simulink model "TST_Tra_Prt"  (R2016b)
settings: Solver=FixedStepDiscrete  StartTime=0.0  StopTime=simTime  FixedStep=sampleTime  RelTol=1e-3
values from neighbouring files (symbols this model uses):
  testCase = 1    [initTST_Tra_Prt_001.m]    (also in initTST_Tra_Prt_002.m = 2; initTST_Tra_Prt_003.m = 3; initTST_Tra_Prt_004.m = 4)
libraries: simulink x9, UnitTest_Lib x4
settings Model: Creator=zhengjinyan  LastModifiedBy=zhengjinyan
settings DebuggingCC: SignalRangeChecking=error

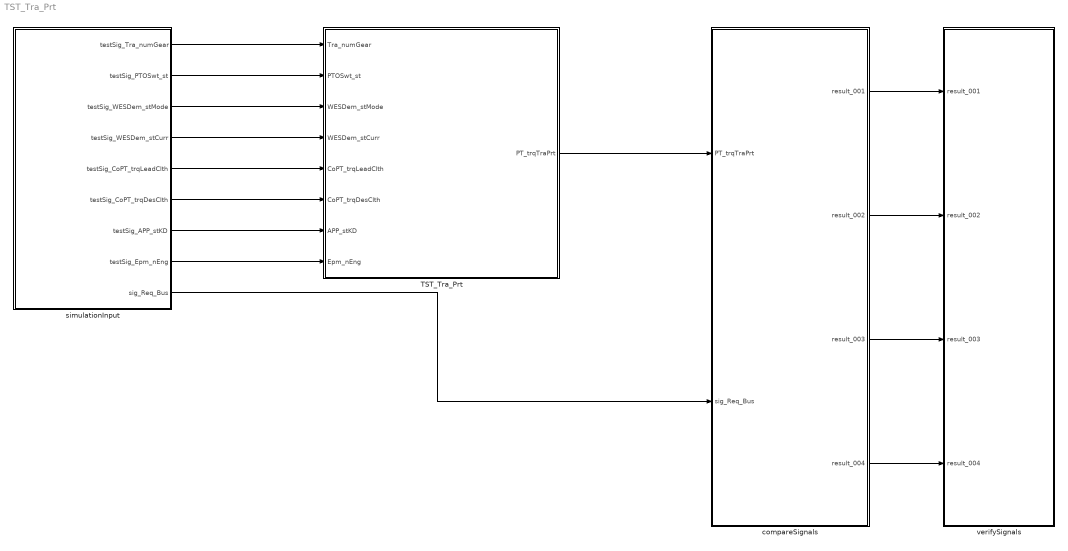
== system TST_Tra_Prt ==
  TST_Tra_Prt : Subsystem
  compareSignals : Subsystem
  simulationInput : Subsystem
  verifySignals : Subsystem
  wires:
  simulationInput/1(testSig_Tra_numGear) -> TST_Tra_Prt/1(Tra_numGear)
  simulationInput/2(testSig_PTOSwt_st) -> TST_Tra_Prt/2(PTOSwt_st)
  simulationInput/3(testSig_WESDem_stMode) -> TST_Tra_Prt/3(WESDem_stMode)
  simulationInput/4(testSig_WESDem_stCurr) -> TST_Tra_Prt/4(WESDem_stCurr)
  simulationInput/5(testSig_CoPT_trqLeadClth) -> TST_Tra_Prt/5(CoPT_trqLeadClth)
  simulationInput/6(testSig_CoPT_trqDesClth) -> TST_Tra_Prt/6(CoPT_trqDesClth)
  simulationInput/7(testSig_APP_stKD) -> TST_Tra_Prt/7(APP_stKD)
  simulationInput/8(testSig_Epm_nEng) -> TST_Tra_Prt/8(Epm_nEng)
  TST_Tra_Prt/1(PT_trqTraPrt) -> compareSignals/1(PT_trqTraPrt)
  simulationInput/9(sig_Req_Bus) -> compareSignals/2(sig_Req_Bus)
  compareSignals/1(result_001) -> verifySignals/1(result_001)
  compareSignals/2(result_002) -> verifySignals/2(result_002)
  compareSignals/3(result_003) -> verifySignals/3(result_003)
  compareSignals/4(result_004) -> verifySignals/4(result_004)

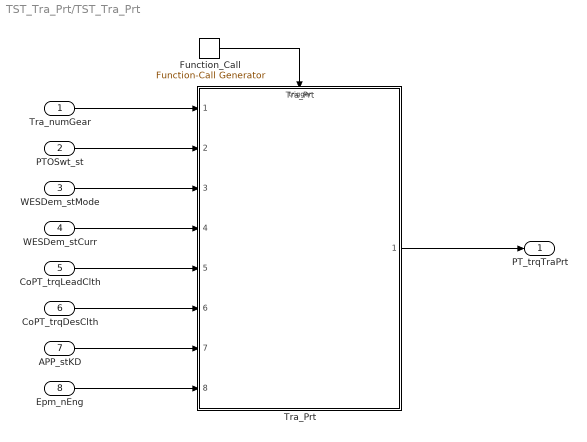
== system TST_Tra_Prt/TST_Tra_Prt ==
  Tra_numGear : Inport
  PTOSwt_st : Inport  Port=2
  WESDem_stMode : Inport  Port=3
  WESDem_stCurr : Inport  Port=4
  CoPT_trqLeadClth : Inport  Port=5
  CoPT_trqDesClth : Inport  Port=6
  APP_stKD : Inport  Port=7
  Epm_nEng : Inport  Port=8
  Function_Call : simulink/Ports & Subsystems/Function-Call Generator  sample_time=sampleTime  numberOfIterations=1
  Tra_Prt : ModelReference  ModelNameDialog=Tra_Prt  SimulationMode=Normal  ModelReferenceVersion=1.31  TriggerPortName=function  TriggerPortTriggerType=function-call  TriggerPortStatesWhenEnabling=held
  PT_trqTraPrt : Outport
  wires:
  Function_Call/1 -> Tra_Prt/Trigger
  Tra_numGear/1 -> Tra_Prt/1
  PTOSwt_st/1 -> Tra_Prt/2
  WESDem_stMode/1 -> Tra_Prt/3
  WESDem_stCurr/1 -> Tra_Prt/4
  CoPT_trqLeadClth/1 -> Tra_Prt/5
  CoPT_trqDesClth/1 -> Tra_Prt/6
  APP_stKD/1 -> Tra_Prt/7
  Epm_nEng/1 -> Tra_Prt/8
  Tra_Prt/1 -> PT_trqTraPrt/1

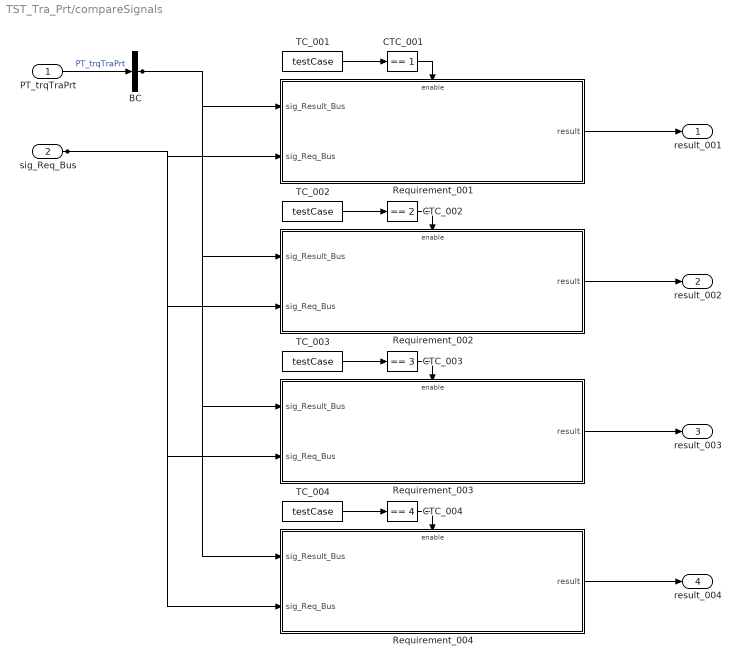
== system TST_Tra_Prt/compareSignals ==
  PT_trqTraPrt : Inport
  sig_Req_Bus : Inport  Port=2
  BC : BusCreator  Inputs=1
  CTC_001 : simulink/Logic and Bit Operations/Compare To Constant  relop===  const=1  OutDataTypeStr=boolean
  CTC_002 : simulink/Logic and Bit Operations/Compare To Constant  relop===  const=2  OutDataTypeStr=boolean
  CTC_003 : simulink/Logic and Bit Operations/Compare To Constant  relop===  const=3  OutDataTypeStr=boolean
  CTC_004 : simulink/Logic and Bit Operations/Compare To Constant  relop===  const=4  OutDataTypeStr=boolean
  Requirement_001 : Subsystem
  Requirement_002 : Subsystem
  Requirement_003 : Subsystem
  Requirement_004 : Subsystem
  TC_001 : Constant  Value=testCase
  TC_002 : Constant  Value=testCase
  TC_003 : Constant  Value=testCase
  TC_004 : Constant  Value=testCase
  result_001 : Outport
  result_002 : Outport  Port=2
  result_003 : Outport  Port=3
  result_004 : Outport  Port=4
  wires:
  PT_trqTraPrt/1 -> BC/1  "PT_trqTraPrt"
  TC_001/1 -> CTC_001/1
  CTC_001/1 -> Requirement_001/Enable
  sig_Req_Bus/1 -> Requirement_001/2(sig_Req_Bus), Requirement_002/2(sig_Req_Bus), Requirement_003/2(sig_Req_Bus), Requirement_004/2(sig_Req_Bus)
  BC/1 -> Requirement_001/1(sig_Result_Bus), Requirement_002/1(sig_Result_Bus), Requirement_003/1(sig_Result_Bus), Requirement_004/1(sig_Result_Bus)
  Requirement_001/1(result) -> result_001/1
  TC_002/1 -> CTC_002/1
  CTC_002/1 -> Requirement_002/Enable
  Requirement_002/1(result) -> result_002/1
  TC_003/1 -> CTC_003/1
  CTC_003/1 -> Requirement_003/Enable
  Requirement_003/1(result) -> result_003/1
  TC_004/1 -> CTC_004/1
  CTC_004/1 -> Requirement_004/Enable
  Requirement_004/1(result) -> result_004/1

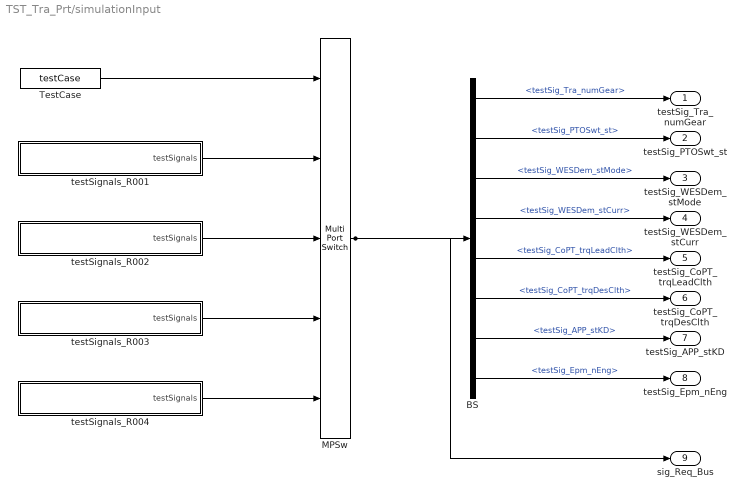
== system TST_Tra_Prt/simulationInput ==
  BS : BusSelector  OutputSignals=testSig_Tra_numGear,testSig_PTOSwt_st,testSig_WESDem_stMode,testSig_WESDem_stCurr,testSig_CoPT_trqLeadClth,testSig_CoPT_trqDesClth,testSig_APP_stKD,testSig_Epm_nEng
  MPSw : MultiPortSwitch  Inputs=4  SaturateOnIntegerOverflow=on  InputSameDT=on
  TestCase : Constant  Value=testCase
  testSignals_R001 : Subsystem
  testSignals_R002 : Subsystem
  testSignals_R003 : Subsystem
  testSignals_R004 : Subsystem
  testSig_Tra_numGear : Outport
  testSig_PTOSwt_st : Outport  Port=2
  testSig_WESDem_stMode : Outport  Port=3
  testSig_WESDem_stCurr : Outport  Port=4
  testSig_CoPT_trqLeadClth : Outport  Port=5
  testSig_CoPT_trqDesClth : Outport  Port=6
  testSig_APP_stKD : Outport  Port=7
  testSig_Epm_nEng : Outport  Port=8
  sig_Req_Bus : Outport  Port=9
  wires:
  BS/1 -> testSig_Tra_numGear/1  "<testSig_Tra_numGear>"
  BS/2 -> testSig_PTOSwt_st/1  "<testSig_PTOSwt_st>"
  BS/3 -> testSig_WESDem_stMode/1  "<testSig_WESDem_stMode>"
  BS/4 -> testSig_WESDem_stCurr/1  "<testSig_WESDem_stCurr>"
  BS/5 -> testSig_CoPT_trqLeadClth/1  "<testSig_CoPT_trqLeadClth>"
  BS/6 -> testSig_CoPT_trqDesClth/1  "<testSig_CoPT_trqDesClth>"
  BS/7 -> testSig_APP_stKD/1  "<testSig_APP_stKD>"
  BS/8 -> testSig_Epm_nEng/1  "<testSig_Epm_nEng>"
  MPSw/1 -> BS/1, sig_Req_Bus/1
  TestCase/1 -> MPSw/1
  testSignals_R001/1(testSignals) -> MPSw/2
  testSignals_R002/1(testSignals) -> MPSw/3
  testSignals_R003/1(testSignals) -> MPSw/4
  testSignals_R004/1(testSignals) -> MPSw/5

== system TST_Tra_Prt/verifySignals ==
  result_001 : Inport
  result_002 : Inport  Port=2
  result_003 : Inport  Port=3
  result_004 : Inport  Port=4
  Assertion_001 : Assertion  Enabled=off
  Assertion_002 : Assertion  Enabled=off
  Assertion_003 : Assertion  Enabled=off
  Assertion_004 : Assertion  Enabled=off
  wires:
  result_001/1 -> Assertion_001/1
  result_002/1 -> Assertion_002/1
  result_003/1 -> Assertion_003/1
  result_004/1 -> Assertion_004/1

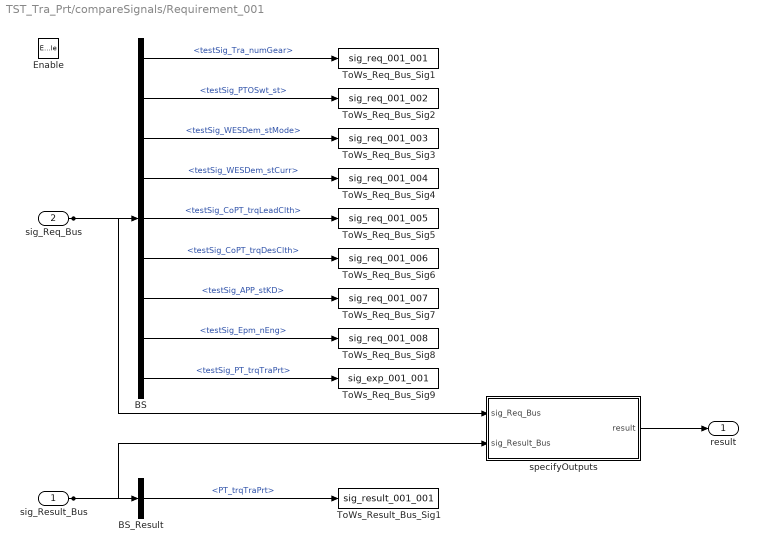
== system TST_Tra_Prt/compareSignals/Requirement_001 ==
  sig_Result_Bus : Inport
  sig_Req_Bus : Inport  Port=2
  Enable : EnablePort
  BS : BusSelector  OutputSignals=testSig_Tra_numGear,testSig_PTOSwt_st,testSig_WESDem_stMode,testSig_WESDem_stCurr,testSig_CoPT_trqLeadClth,testSig_CoPT_trqDesClth,testSig_APP_stKD,testSig_Epm_nEng,testSig_PT_trqTraPrt
  BS_Result : BusSelector  OutputSignals=PT_trqTraPrt
  ToWs_Req_Bus_Sig1 : ToWorkspace  VariableName=sig_req_001_001  SaveFormat=Structure With Time
  ToWs_Req_Bus_Sig2 : ToWorkspace  VariableName=sig_req_001_002  SaveFormat=Structure With Time
  ToWs_Req_Bus_Sig3 : ToWorkspace  VariableName=sig_req_001_003  SaveFormat=Structure With Time
  ToWs_Req_Bus_Sig4 : ToWorkspace  VariableName=sig_req_001_004  SaveFormat=Structure With Time
  ToWs_Req_Bus_Sig5 : ToWorkspace  VariableName=sig_req_001_005  SaveFormat=Structure With Time
  ToWs_Req_Bus_Sig6 : ToWorkspace  VariableName=sig_req_001_006  SaveFormat=Structure With Time
  ToWs_Req_Bus_Sig7 : ToWorkspace  VariableName=sig_req_001_007  SaveFormat=Structure With Time
  ToWs_Req_Bus_Sig8 : ToWorkspace  VariableName=sig_req_001_008  SaveFormat=Structure With Time
  ToWs_Req_Bus_Sig9 : ToWorkspace  VariableName=sig_exp_001_001  SaveFormat=Structure With Time
  ToWs_Result_Bus_Sig1 : ToWorkspace  VariableName=sig_result_001_001  SaveFormat=Structure With Time
  specifyOutputs : Subsystem
  result : Outport
  wires:
  sig_Req_Bus/1 -> BS/1, specifyOutputs/1(sig_Req_Bus)
  BS/1 -> ToWs_Req_Bus_Sig1/1  "<testSig_Tra_numGear>"
  BS/2 -> ToWs_Req_Bus_Sig2/1  "<testSig_PTOSwt_st>"
  BS/3 -> ToWs_Req_Bus_Sig3/1  "<testSig_WESDem_stMode>"
  BS/4 -> ToWs_Req_Bus_Sig4/1  "<testSig_WESDem_stCurr>"
  BS/5 -> ToWs_Req_Bus_Sig5/1  "<testSig_CoPT_trqLeadClth>"
  BS/6 -> ToWs_Req_Bus_Sig6/1  "<testSig_CoPT_trqDesClth>"
  BS/7 -> ToWs_Req_Bus_Sig7/1  "<testSig_APP_stKD>"
  BS/8 -> ToWs_Req_Bus_Sig8/1  "<testSig_Epm_nEng>"
  BS/9 -> ToWs_Req_Bus_Sig9/1  "<testSig_PT_trqTraPrt>"
  sig_Result_Bus/1 -> BS_Result/1, specifyOutputs/2(sig_Result_Bus)
  BS_Result/1 -> ToWs_Result_Bus_Sig1/1  "<PT_trqTraPrt>"
  specifyOutputs/1(result) -> result/1

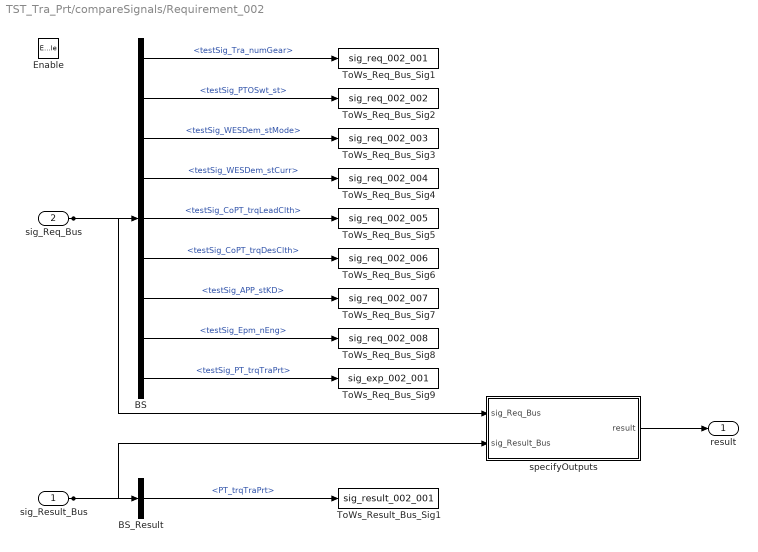
== system TST_Tra_Prt/compareSignals/Requirement_002 ==
  sig_Result_Bus : Inport
  sig_Req_Bus : Inport  Port=2
  Enable : EnablePort
  BS : BusSelector  OutputSignals=testSig_Tra_numGear,testSig_PTOSwt_st,testSig_WESDem_stMode,testSig_WESDem_stCurr,testSig_CoPT_trqLeadClth,testSig_CoPT_trqDesClth,testSig_APP_stKD,testSig_Epm_nEng,testSig_PT_trqTraPrt
  BS_Result : BusSelector  OutputSignals=PT_trqTraPrt
  ToWs_Req_Bus_Sig1 : ToWorkspace  VariableName=sig_req_002_001  SaveFormat=Structure With Time
  ToWs_Req_Bus_Sig2 : ToWorkspace  VariableName=sig_req_002_002  SaveFormat=Structure With Time
  ToWs_Req_Bus_Sig3 : ToWorkspace  VariableName=sig_req_002_003  SaveFormat=Structure With Time
  ToWs_Req_Bus_Sig4 : ToWorkspace  VariableName=sig_req_002_004  SaveFormat=Structure With Time
  ToWs_Req_Bus_Sig5 : ToWorkspace  VariableName=sig_req_002_005  SaveFormat=Structure With Time
  ToWs_Req_Bus_Sig6 : ToWorkspace  VariableName=sig_req_002_006  SaveFormat=Structure With Time
  ToWs_Req_Bus_Sig7 : ToWorkspace  VariableName=sig_req_002_007  SaveFormat=Structure With Time
  ToWs_Req_Bus_Sig8 : ToWorkspace  VariableName=sig_req_002_008  SaveFormat=Structure With Time
  ToWs_Req_Bus_Sig9 : ToWorkspace  VariableName=sig_exp_002_001  SaveFormat=Structure With Time
  ToWs_Result_Bus_Sig1 : ToWorkspace  VariableName=sig_result_002_001  SaveFormat=Structure With Time
  specifyOutputs : Subsystem
  result : Outport
  wires:
  sig_Req_Bus/1 -> BS/1, specifyOutputs/1(sig_Req_Bus)
  BS/1 -> ToWs_Req_Bus_Sig1/1  "<testSig_Tra_numGear>"
  BS/2 -> ToWs_Req_Bus_Sig2/1  "<testSig_PTOSwt_st>"
  BS/3 -> ToWs_Req_Bus_Sig3/1  "<testSig_WESDem_stMode>"
  BS/4 -> ToWs_Req_Bus_Sig4/1  "<testSig_WESDem_stCurr>"
  BS/5 -> ToWs_Req_Bus_Sig5/1  "<testSig_CoPT_trqLeadClth>"
  BS/6 -> ToWs_Req_Bus_Sig6/1  "<testSig_CoPT_trqDesClth>"
  BS/7 -> ToWs_Req_Bus_Sig7/1  "<testSig_APP_stKD>"
  BS/8 -> ToWs_Req_Bus_Sig8/1  "<testSig_Epm_nEng>"
  BS/9 -> ToWs_Req_Bus_Sig9/1  "<testSig_PT_trqTraPrt>"
  sig_Result_Bus/1 -> BS_Result/1, specifyOutputs/2(sig_Result_Bus)
  BS_Result/1 -> ToWs_Result_Bus_Sig1/1  "<PT_trqTraPrt>"
  specifyOutputs/1(result) -> result/1

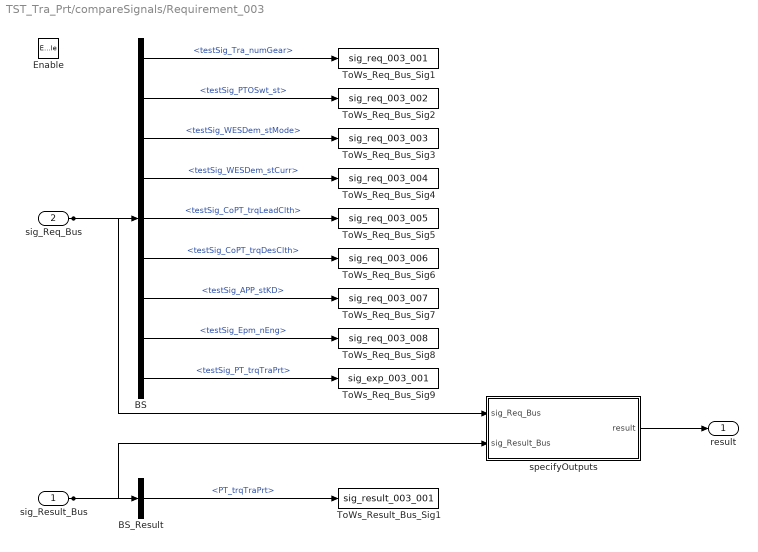
== system TST_Tra_Prt/compareSignals/Requirement_003 ==
  sig_Result_Bus : Inport
  sig_Req_Bus : Inport  Port=2
  Enable : EnablePort
  BS : BusSelector  OutputSignals=testSig_Tra_numGear,testSig_PTOSwt_st,testSig_WESDem_stMode,testSig_WESDem_stCurr,testSig_CoPT_trqLeadClth,testSig_CoPT_trqDesClth,testSig_APP_stKD,testSig_Epm_nEng,testSig_PT_trqTraPrt
  BS_Result : BusSelector  OutputSignals=PT_trqTraPrt
  ToWs_Req_Bus_Sig1 : ToWorkspace  VariableName=sig_req_003_001  SaveFormat=Structure With Time
  ToWs_Req_Bus_Sig2 : ToWorkspace  VariableName=sig_req_003_002  SaveFormat=Structure With Time
  ToWs_Req_Bus_Sig3 : ToWorkspace  VariableName=sig_req_003_003  SaveFormat=Structure With Time
  ToWs_Req_Bus_Sig4 : ToWorkspace  VariableName=sig_req_003_004  SaveFormat=Structure With Time
  ToWs_Req_Bus_Sig5 : ToWorkspace  VariableName=sig_req_003_005  SaveFormat=Structure With Time
  ToWs_Req_Bus_Sig6 : ToWorkspace  VariableName=sig_req_003_006  SaveFormat=Structure With Time
  ToWs_Req_Bus_Sig7 : ToWorkspace  VariableName=sig_req_003_007  SaveFormat=Structure With Time
  ToWs_Req_Bus_Sig8 : ToWorkspace  VariableName=sig_req_003_008  SaveFormat=Structure With Time
  ToWs_Req_Bus_Sig9 : ToWorkspace  VariableName=sig_exp_003_001  SaveFormat=Structure With Time
  ToWs_Result_Bus_Sig1 : ToWorkspace  VariableName=sig_result_003_001  SaveFormat=Structure With Time
  specifyOutputs : Subsystem
  result : Outport
  wires:
  sig_Req_Bus/1 -> BS/1, specifyOutputs/1(sig_Req_Bus)
  BS/1 -> ToWs_Req_Bus_Sig1/1  "<testSig_Tra_numGear>"
  BS/2 -> ToWs_Req_Bus_Sig2/1  "<testSig_PTOSwt_st>"
  BS/3 -> ToWs_Req_Bus_Sig3/1  "<testSig_WESDem_stMode>"
  BS/4 -> ToWs_Req_Bus_Sig4/1  "<testSig_WESDem_stCurr>"
  BS/5 -> ToWs_Req_Bus_Sig5/1  "<testSig_CoPT_trqLeadClth>"
  BS/6 -> ToWs_Req_Bus_Sig6/1  "<testSig_CoPT_trqDesClth>"
  BS/7 -> ToWs_Req_Bus_Sig7/1  "<testSig_APP_stKD>"
  BS/8 -> ToWs_Req_Bus_Sig8/1  "<testSig_Epm_nEng>"
  BS/9 -> ToWs_Req_Bus_Sig9/1  "<testSig_PT_trqTraPrt>"
  sig_Result_Bus/1 -> BS_Result/1, specifyOutputs/2(sig_Result_Bus)
  BS_Result/1 -> ToWs_Result_Bus_Sig1/1  "<PT_trqTraPrt>"
  specifyOutputs/1(result) -> result/1

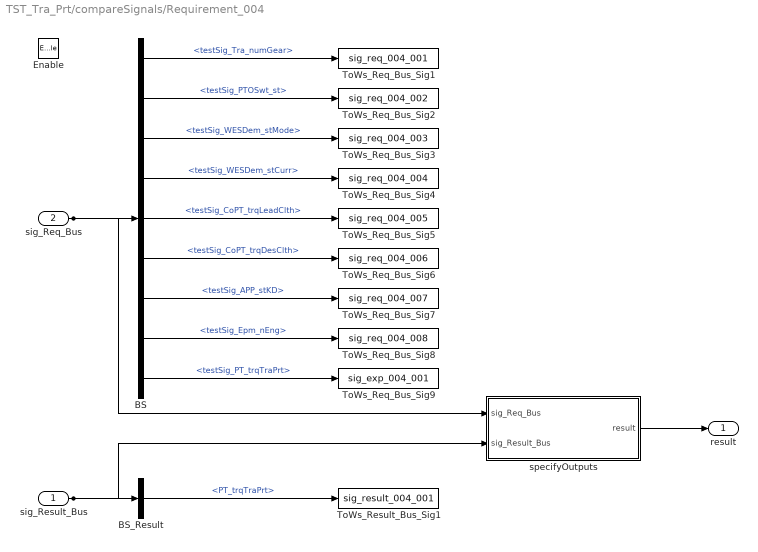
== system TST_Tra_Prt/compareSignals/Requirement_004 ==
  sig_Result_Bus : Inport
  sig_Req_Bus : Inport  Port=2
  Enable : EnablePort
  BS : BusSelector  OutputSignals=testSig_Tra_numGear,testSig_PTOSwt_st,testSig_WESDem_stMode,testSig_WESDem_stCurr,testSig_CoPT_trqLeadClth,testSig_CoPT_trqDesClth,testSig_APP_stKD,testSig_Epm_nEng,testSig_PT_trqTraPrt
  BS_Result : BusSelector  OutputSignals=PT_trqTraPrt
  ToWs_Req_Bus_Sig1 : ToWorkspace  VariableName=sig_req_004_001  SaveFormat=Structure With Time
  ToWs_Req_Bus_Sig2 : ToWorkspace  VariableName=sig_req_004_002  SaveFormat=Structure With Time
  ToWs_Req_Bus_Sig3 : ToWorkspace  VariableName=sig_req_004_003  SaveFormat=Structure With Time
  ToWs_Req_Bus_Sig4 : ToWorkspace  VariableName=sig_req_004_004  SaveFormat=Structure With Time
  ToWs_Req_Bus_Sig5 : ToWorkspace  VariableName=sig_req_004_005  SaveFormat=Structure With Time
  ToWs_Req_Bus_Sig6 : ToWorkspace  VariableName=sig_req_004_006  SaveFormat=Structure With Time
  ToWs_Req_Bus_Sig7 : ToWorkspace  VariableName=sig_req_004_007  SaveFormat=Structure With Time
  ToWs_Req_Bus_Sig8 : ToWorkspace  VariableName=sig_req_004_008  SaveFormat=Structure With Time
  ToWs_Req_Bus_Sig9 : ToWorkspace  VariableName=sig_exp_004_001  SaveFormat=Structure With Time
  ToWs_Result_Bus_Sig1 : ToWorkspace  VariableName=sig_result_004_001  SaveFormat=Structure With Time
  specifyOutputs : Subsystem
  result : Outport
  wires:
  sig_Req_Bus/1 -> BS/1, specifyOutputs/1(sig_Req_Bus)
  BS/1 -> ToWs_Req_Bus_Sig1/1  "<testSig_Tra_numGear>"
  BS/2 -> ToWs_Req_Bus_Sig2/1  "<testSig_PTOSwt_st>"
  BS/3 -> ToWs_Req_Bus_Sig3/1  "<testSig_WESDem_stMode>"
  BS/4 -> ToWs_Req_Bus_Sig4/1  "<testSig_WESDem_stCurr>"
  BS/5 -> ToWs_Req_Bus_Sig5/1  "<testSig_CoPT_trqLeadClth>"
  BS/6 -> ToWs_Req_Bus_Sig6/1  "<testSig_CoPT_trqDesClth>"
  BS/7 -> ToWs_Req_Bus_Sig7/1  "<testSig_APP_stKD>"
  BS/8 -> ToWs_Req_Bus_Sig8/1  "<testSig_Epm_nEng>"
  BS/9 -> ToWs_Req_Bus_Sig9/1  "<testSig_PT_trqTraPrt>"
  sig_Result_Bus/1 -> BS_Result/1, specifyOutputs/2(sig_Result_Bus)
  BS_Result/1 -> ToWs_Result_Bus_Sig1/1  "<PT_trqTraPrt>"
  specifyOutputs/1(result) -> result/1

== system TST_Tra_Prt/simulationInput/testSignals_R001 ==
  BC : BusCreator  Inputs=9
  spec_APP_stKD : FromWorkspace  VariableName=testSig_APP_stKD  Interpolate=off  OutputAfterFinalValue=Holding final value
  spec_CoPT_trqDesClth : FromWorkspace  VariableName=testSig_CoPT_trqDesClth  Interpolate=off  OutputAfterFinalValue=Holding final value
  spec_CoPT_trqLeadClth : FromWorkspace  VariableName=testSig_CoPT_trqLeadClth  Interpolate=off  OutputAfterFinalValue=Holding final value
  spec_Epm_nEng : FromWorkspace  VariableName=testSig_Epm_nEng  Interpolate=off  OutputAfterFinalValue=Holding final value
  spec_PTOSwt_st : FromWorkspace  VariableName=testSig_PTOSwt_st  Interpolate=off  OutputAfterFinalValue=Holding final value
  spec_PT_trqTraPrt : FromWorkspace  VariableName=testSig_PT_trqTraPrt  Interpolate=off  OutputAfterFinalValue=Holding final value
  spec_Tra_numGear : FromWorkspace  VariableName=testSig_Tra_numGear  Interpolate=off  OutputAfterFinalValue=Holding final value
  spec_WESDem_stCurr : FromWorkspace  VariableName=testSig_WESDem_stCurr  Interpolate=off  OutputAfterFinalValue=Holding final value
  spec_WESDem_stMode : FromWorkspace  VariableName=testSig_WESDem_stMode  Interpolate=off  OutputAfterFinalValue=Holding final value
  testSignals : Outport
  wires:
  BC/1 -> testSignals/1
  spec_Tra_numGear/1 -> BC/1  "testSig_Tra_numGear"
  spec_PTOSwt_st/1 -> BC/2  "testSig_PTOSwt_st"
  spec_WESDem_stMode/1 -> BC/3  "testSig_WESDem_stMode"
  spec_WESDem_stCurr/1 -> BC/4  "testSig_WESDem_stCurr"
  spec_CoPT_trqLeadClth/1 -> BC/5  "testSig_CoPT_trqLeadClth"
  spec_CoPT_trqDesClth/1 -> BC/6  "testSig_CoPT_trqDesClth"
  spec_APP_stKD/1 -> BC/7  "testSig_APP_stKD"
  spec_Epm_nEng/1 -> BC/8  "testSig_Epm_nEng"
  spec_PT_trqTraPrt/1 -> BC/9  "testSig_PT_trqTraPrt"

== system TST_Tra_Prt/simulationInput/testSignals_R002 ==
  BC : BusCreator  Inputs=9
  spec_APP_stKD : FromWorkspace  VariableName=testSig_APP_stKD  Interpolate=off  OutputAfterFinalValue=Holding final value
  spec_CoPT_trqDesClth : FromWorkspace  VariableName=testSig_CoPT_trqDesClth  Interpolate=off  OutputAfterFinalValue=Holding final value
  spec_CoPT_trqLeadClth : FromWorkspace  VariableName=testSig_CoPT_trqLeadClth  Interpolate=off  OutputAfterFinalValue=Holding final value
  spec_Epm_nEng : FromWorkspace  VariableName=testSig_Epm_nEng  Interpolate=off  OutputAfterFinalValue=Holding final value
  spec_PTOSwt_st : FromWorkspace  VariableName=testSig_PTOSwt_st  Interpolate=off  OutputAfterFinalValue=Holding final value
  spec_PT_trqTraPrt : FromWorkspace  VariableName=testSig_PT_trqTraPrt  Interpolate=off  OutputAfterFinalValue=Holding final value
  spec_Tra_numGear : FromWorkspace  VariableName=testSig_Tra_numGear  Interpolate=off  OutputAfterFinalValue=Holding final value
  spec_WESDem_stCurr : FromWorkspace  VariableName=testSig_WESDem_stCurr  Interpolate=off  OutputAfterFinalValue=Holding final value
  spec_WESDem_stMode : FromWorkspace  VariableName=testSig_WESDem_stMode  Interpolate=off  OutputAfterFinalValue=Holding final value
  testSignals : Outport
  wires:
  BC/1 -> testSignals/1
  spec_Tra_numGear/1 -> BC/1  "testSig_Tra_numGear"
  spec_PTOSwt_st/1 -> BC/2  "testSig_PTOSwt_st"
  spec_WESDem_stMode/1 -> BC/3  "testSig_WESDem_stMode"
  spec_WESDem_stCurr/1 -> BC/4  "testSig_WESDem_stCurr"
  spec_CoPT_trqLeadClth/1 -> BC/5  "testSig_CoPT_trqLeadClth"
  spec_CoPT_trqDesClth/1 -> BC/6  "testSig_CoPT_trqDesClth"
  spec_APP_stKD/1 -> BC/7  "testSig_APP_stKD"
  spec_Epm_nEng/1 -> BC/8  "testSig_Epm_nEng"
  spec_PT_trqTraPrt/1 -> BC/9  "testSig_PT_trqTraPrt"

== system TST_Tra_Prt/simulationInput/testSignals_R003 ==
  BC : BusCreator  Inputs=9
  spec_APP_stKD : FromWorkspace  VariableName=testSig_APP_stKD  Interpolate=off  OutputAfterFinalValue=Holding final value
  spec_CoPT_trqDesClth : FromWorkspace  VariableName=testSig_CoPT_trqDesClth  Interpolate=off  OutputAfterFinalValue=Holding final value
  spec_CoPT_trqLeadClth : FromWorkspace  VariableName=testSig_CoPT_trqLeadClth  Interpolate=off  OutputAfterFinalValue=Holding final value
  spec_Epm_nEng : FromWorkspace  VariableName=testSig_Epm_nEng  Interpolate=off  OutputAfterFinalValue=Holding final value
  spec_PTOSwt_st : FromWorkspace  VariableName=testSig_PTOSwt_st  Interpolate=off  OutputAfterFinalValue=Holding final value
  spec_PT_trqTraPrt : FromWorkspace  VariableName=testSig_PT_trqTraPrt  Interpolate=off  OutputAfterFinalValue=Holding final value
  spec_Tra_numGear : FromWorkspace  VariableName=testSig_Tra_numGear  Interpolate=off  OutputAfterFinalValue=Holding final value
  spec_WESDem_stCurr : FromWorkspace  VariableName=testSig_WESDem_stCurr  Interpolate=off  OutputAfterFinalValue=Holding final value
  spec_WESDem_stMode : FromWorkspace  VariableName=testSig_WESDem_stMode  Interpolate=off  OutputAfterFinalValue=Holding final value
  testSignals : Outport
  wires:
  BC/1 -> testSignals/1
  spec_Tra_numGear/1 -> BC/1  "testSig_Tra_numGear"
  spec_PTOSwt_st/1 -> BC/2  "testSig_PTOSwt_st"
  spec_WESDem_stMode/1 -> BC/3  "testSig_WESDem_stMode"
  spec_WESDem_stCurr/1 -> BC/4  "testSig_WESDem_stCurr"
  spec_CoPT_trqLeadClth/1 -> BC/5  "testSig_CoPT_trqLeadClth"
  spec_CoPT_trqDesClth/1 -> BC/6  "testSig_CoPT_trqDesClth"
  spec_APP_stKD/1 -> BC/7  "testSig_APP_stKD"
  spec_Epm_nEng/1 -> BC/8  "testSig_Epm_nEng"
  spec_PT_trqTraPrt/1 -> BC/9  "testSig_PT_trqTraPrt"

== system TST_Tra_Prt/simulationInput/testSignals_R004 ==
  BC : BusCreator  Inputs=9
  spec_APP_stKD : FromWorkspace  VariableName=testSig_APP_stKD  Interpolate=off  OutputAfterFinalValue=Holding final value
  spec_CoPT_trqDesClth : FromWorkspace  VariableName=testSig_CoPT_trqDesClth  Interpolate=off  OutputAfterFinalValue=Holding final value
  spec_CoPT_trqLeadClth : FromWorkspace  VariableName=testSig_CoPT_trqLeadClth  Interpolate=off  OutputAfterFinalValue=Holding final value
  spec_Epm_nEng : FromWorkspace  VariableName=testSig_Epm_nEng  Interpolate=off  OutputAfterFinalValue=Holding final value
  spec_PTOSwt_st : FromWorkspace  VariableName=testSig_PTOSwt_st  Interpolate=off  OutputAfterFinalValue=Holding final value
  spec_PT_trqTraPrt : FromWorkspace  VariableName=testSig_PT_trqTraPrt  Interpolate=off  OutputAfterFinalValue=Holding final value
  spec_Tra_numGear : FromWorkspace  VariableName=testSig_Tra_numGear  Interpolate=off  OutputAfterFinalValue=Holding final value
  spec_WESDem_stCurr : FromWorkspace  VariableName=testSig_WESDem_stCurr  Interpolate=off  OutputAfterFinalValue=Holding final value
  spec_WESDem_stMode : FromWorkspace  VariableName=testSig_WESDem_stMode  Interpolate=off  OutputAfterFinalValue=Holding final value
  testSignals : Outport
  wires:
  BC/1 -> testSignals/1
  spec_Tra_numGear/1 -> BC/1  "testSig_Tra_numGear"
  spec_PTOSwt_st/1 -> BC/2  "testSig_PTOSwt_st"
  spec_WESDem_stMode/1 -> BC/3  "testSig_WESDem_stMode"
  spec_WESDem_stCurr/1 -> BC/4  "testSig_WESDem_stCurr"
  spec_CoPT_trqLeadClth/1 -> BC/5  "testSig_CoPT_trqLeadClth"
  spec_CoPT_trqDesClth/1 -> BC/6  "testSig_CoPT_trqDesClth"
  spec_APP_stKD/1 -> BC/7  "testSig_APP_stKD"
  spec_Epm_nEng/1 -> BC/8  "testSig_Epm_nEng"
  spec_PT_trqTraPrt/1 -> BC/9  "testSig_PT_trqTraPrt"

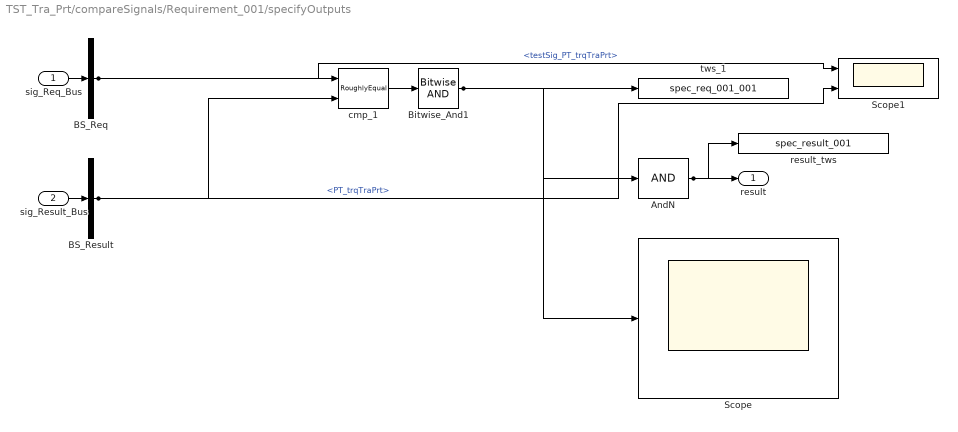
== system TST_Tra_Prt/compareSignals/Requirement_001/specifyOutputs ==
  sig_Req_Bus : Inport
  sig_Result_Bus : Inport  Port=2
  AndN : Logic  Inputs=1
  BS_Req : BusSelector  OutputSignals=testSig_PT_trqTraPrt
  BS_Result : BusSelector  OutputSignals=PT_trqTraPrt
  Bitwise_And1 : simulink/Logic and Bit Operations/Bitwise Operator  logicop=AND  UseBitMask=off  BitMask=bin2dec('11011001')  BitMaskRealWorld=Stored Integer
  Scope : Scope
  Scope1 : Scope  NumInputPorts=2
  cmp_1 : UnitTest_Lib/RoughlyEqual  slope=0.1
  result_tws : ToWorkspace  VariableName=spec_result_001
  tws_1 : ToWorkspace  VariableName=spec_req_001_001
  result : Outport
  wires:
  sig_Req_Bus/1 -> BS_Req/1
  sig_Result_Bus/1 -> BS_Result/1
  AndN/1 -> result/1, result_tws/1
  BS_Req/1 -> cmp_1/1, Scope1/1  "<testSig_PT_trqTraPrt>"
  BS_Result/1 -> cmp_1/2, Scope1/2  "<PT_trqTraPrt>"
  cmp_1/1 -> Bitwise_And1/1
  Bitwise_And1/1 -> tws_1/1, AndN/1, Scope/1

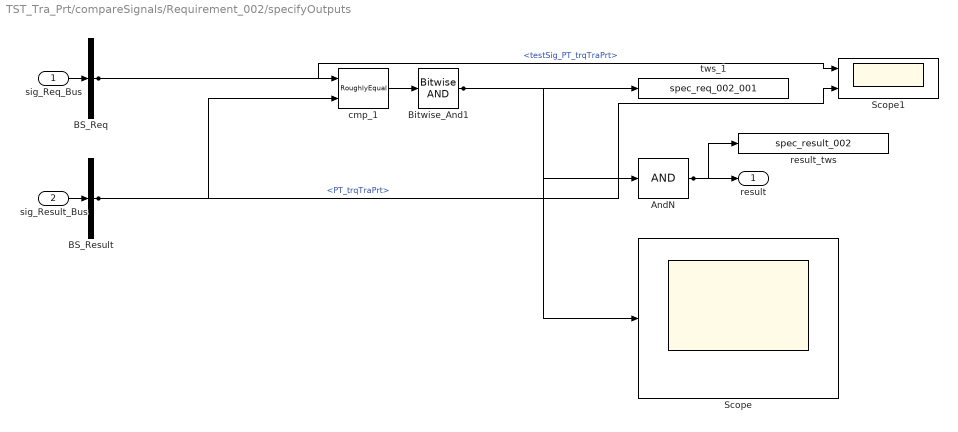
== system TST_Tra_Prt/compareSignals/Requirement_002/specifyOutputs ==
  sig_Req_Bus : Inport
  sig_Result_Bus : Inport  Port=2
  AndN : Logic  Inputs=1
  BS_Req : BusSelector  OutputSignals=testSig_PT_trqTraPrt
  BS_Result : BusSelector  OutputSignals=PT_trqTraPrt
  Bitwise_And1 : simulink/Logic and Bit Operations/Bitwise Operator  logicop=AND  UseBitMask=off  BitMask=bin2dec('11011001')  BitMaskRealWorld=Stored Integer
  Scope : Scope
  Scope1 : Scope  NumInputPorts=2
  cmp_1 : UnitTest_Lib/RoughlyEqual  slope=0.1
  result_tws : ToWorkspace  VariableName=spec_result_002
  tws_1 : ToWorkspace  VariableName=spec_req_002_001
  result : Outport
  wires:
  sig_Req_Bus/1 -> BS_Req/1
  sig_Result_Bus/1 -> BS_Result/1
  AndN/1 -> result/1, result_tws/1
  BS_Req/1 -> cmp_1/1, Scope1/1  "<testSig_PT_trqTraPrt>"
  BS_Result/1 -> cmp_1/2, Scope1/2  "<PT_trqTraPrt>"
  cmp_1/1 -> Bitwise_And1/1
  Bitwise_And1/1 -> tws_1/1, AndN/1, Scope/1

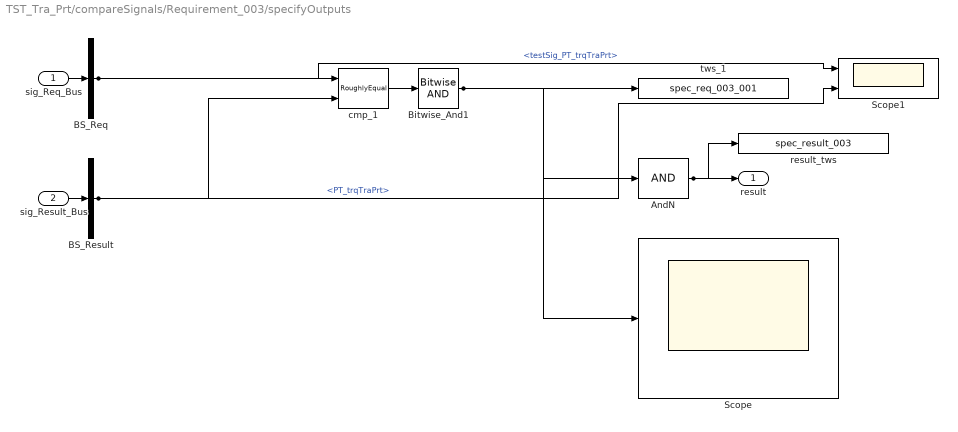
== system TST_Tra_Prt/compareSignals/Requirement_003/specifyOutputs ==
  sig_Req_Bus : Inport
  sig_Result_Bus : Inport  Port=2
  AndN : Logic  Inputs=1
  BS_Req : BusSelector  OutputSignals=testSig_PT_trqTraPrt
  BS_Result : BusSelector  OutputSignals=PT_trqTraPrt
  Bitwise_And1 : simulink/Logic and Bit Operations/Bitwise Operator  logicop=AND  UseBitMask=off  BitMask=bin2dec('11011001')  BitMaskRealWorld=Stored Integer
  Scope : Scope
  Scope1 : Scope  NumInputPorts=2
  cmp_1 : UnitTest_Lib/RoughlyEqual  slope=0.1
  result_tws : ToWorkspace  VariableName=spec_result_003
  tws_1 : ToWorkspace  VariableName=spec_req_003_001
  result : Outport
  wires:
  sig_Req_Bus/1 -> BS_Req/1
  sig_Result_Bus/1 -> BS_Result/1
  AndN/1 -> result/1, result_tws/1
  BS_Req/1 -> cmp_1/1, Scope1/1  "<testSig_PT_trqTraPrt>"
  BS_Result/1 -> cmp_1/2, Scope1/2  "<PT_trqTraPrt>"
  cmp_1/1 -> Bitwise_And1/1
  Bitwise_And1/1 -> tws_1/1, AndN/1, Scope/1

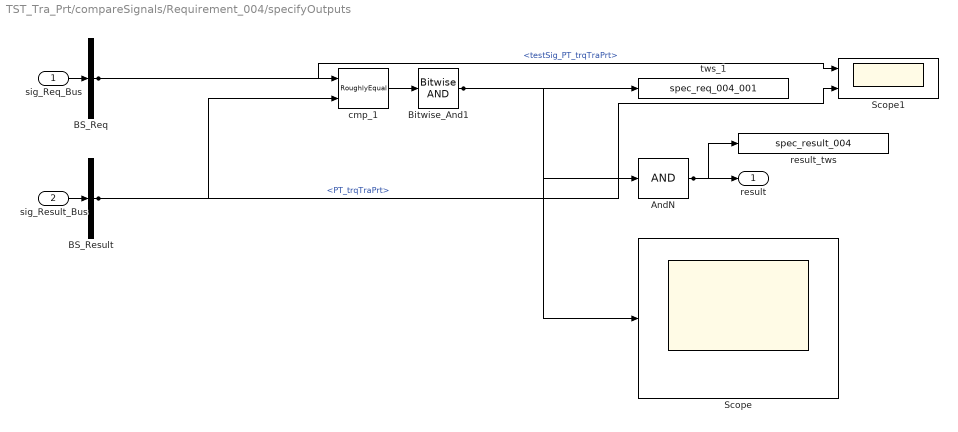
== system TST_Tra_Prt/compareSignals/Requirement_004/specifyOutputs ==
  sig_Req_Bus : Inport
  sig_Result_Bus : Inport  Port=2
  AndN : Logic  Inputs=1
  BS_Req : BusSelector  OutputSignals=testSig_PT_trqTraPrt
  BS_Result : BusSelector  OutputSignals=PT_trqTraPrt
  Bitwise_And1 : simulink/Logic and Bit Operations/Bitwise Operator  logicop=AND  UseBitMask=off  BitMask=bin2dec('11011001')  BitMaskRealWorld=Stored Integer
  Scope : Scope
  Scope1 : Scope  NumInputPorts=2
  cmp_1 : UnitTest_Lib/RoughlyEqual  slope=0.1
  result_tws : ToWorkspace  VariableName=spec_result_004
  tws_1 : ToWorkspace  VariableName=spec_req_004_001
  result : Outport
  wires:
  sig_Req_Bus/1 -> BS_Req/1
  sig_Result_Bus/1 -> BS_Result/1
  AndN/1 -> result/1, result_tws/1
  BS_Req/1 -> cmp_1/1, Scope1/1  "<testSig_PT_trqTraPrt>"
  BS_Result/1 -> cmp_1/2, Scope1/2  "<PT_trqTraPrt>"
  cmp_1/1 -> Bitwise_And1/1
  Bitwise_And1/1 -> tws_1/1, AndN/1, Scope/1
